simulink model "pneumatiques"  (R2024b)
settings: Solver=VariableStepAuto  StartTime=0.0  StopTime=10.0  RelTol=1e-3
settings Model: Creator=marti  LastModifiedBy=marti

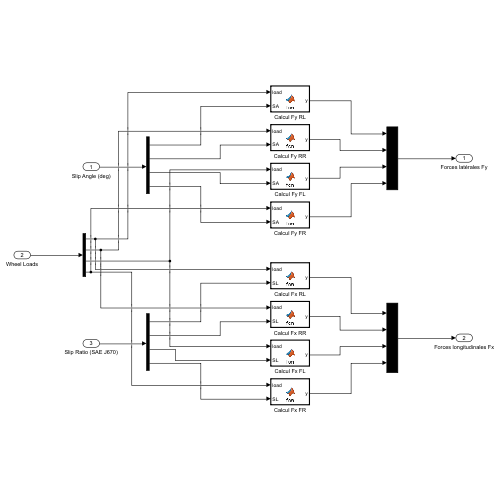
[thumbnail: Simulink's stored preview of the top-level diagram]
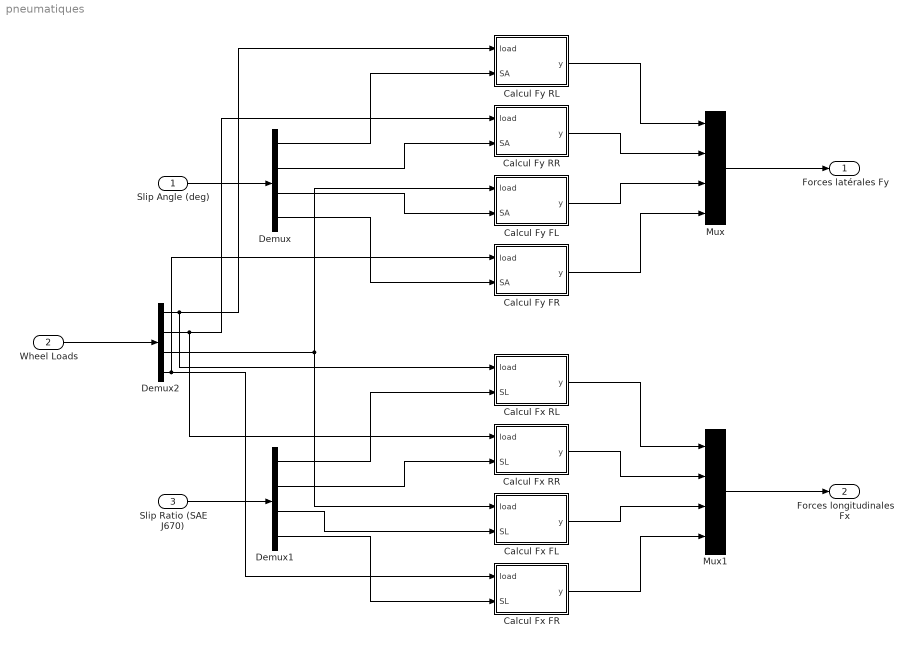
== system pneumatiques ==
  Slip Angle (deg) : Inport
  Wheel Loads : Inport  Port=2
  Slip Ratio (SAE J670) : Inport  Port=3
  Calcul Fx FL : MATLAB Function  TreatAsAtomicUnit=on
  Calcul Fx FR : MATLAB Function  TreatAsAtomicUnit=on
  Calcul Fx RL : MATLAB Function  TreatAsAtomicUnit=on
  Calcul Fx RR : MATLAB Function  TreatAsAtomicUnit=on
  Calcul Fy FL : MATLAB Function  TreatAsAtomicUnit=on
  Calcul Fy FR : MATLAB Function  TreatAsAtomicUnit=on
  Calcul Fy RL : MATLAB Function  TreatAsAtomicUnit=on
  Calcul Fy RR : MATLAB Function  TreatAsAtomicUnit=on
  Demux : Demux
  Demux1 : Demux
  Demux2 : Demux
  Mux : Mux
  Mux1 : Mux
  Forces latérales Fy : Outport
  Forces longitudinales Fx : Outport  Port=2
  wires:
  Slip Angle (deg)/1 -> Demux/1
  Demux/1 -> Calcul Fy RL/2(SA)
  Demux/2 -> Calcul Fy RR/2(SA)
  Demux/3 -> Calcul Fy FL/2(SA)
  Demux/4 -> Calcul Fy FR/2(SA)
  Slip Ratio (SAE J670)/1 -> Demux1/1
  Demux1/2 -> Calcul Fx RR/2(SL)
  Demux1/4 -> Calcul Fx FR/2(SL)
  Demux1/1 -> Calcul Fx RL/2(SL)
  Demux1/3 -> Calcul Fx FL/2(SL)
  Wheel Loads/1 -> Demux2/1
  Demux2/1 -> Calcul Fx RL/1(load), Calcul Fy RL/1(load)
  Demux2/2 -> Calcul Fx RR/1(load), Calcul Fy RR/1(load)
  Demux2/3 -> Calcul Fy FL/1(load), Calcul Fx FL/1(load)
  Demux2/4 -> Calcul Fx FR/1(load), Calcul Fy FR/1(load)
  Calcul Fy RL/1(y) -> Mux/1
  Calcul Fy RR/1(y) -> Mux/2
  Calcul Fy FL/1(y) -> Mux/3
  Calcul Fy FR/1(y) -> Mux/4
  Calcul Fx RL/1(y) -> Mux1/1
  Calcul Fx RR/1(y) -> Mux1/2
  Calcul Fx FL/1(y) -> Mux1/3
  Calcul Fx FR/1(y) -> Mux1/4
  Mux1/1 -> Forces longitudinales Fx/1
  Mux/1 -> Forces latérales Fy/1

== matlab function pneumatiques/Calcul Fy RL ==
  data: load input; y output; SA input
function y = fcn(load,SA)

y = fonction_pacejka_3D_SA(load,SA);
end

== matlab function pneumatiques/Calcul Fy FR ==
  data: load input; y output; SA input
function y = fcn(load,SA)

y = fonction_pacejka_3D_SA(load,SA);
end

== matlab function pneumatiques/Calcul Fy FL ==
  data: load input; y output; SA input
function y = fcn(load,SA)

y = fonction_pacejka_3D_SA(load,SA);
end

== matlab function pneumatiques/Calcul Fx FL ==
  data: load input; y output; SL input
function y = fcn(load,SL)

y = fonction_pacejka_3D_SL(load,SL);
end

== matlab function pneumatiques/Calcul Fx FR ==
  data: load input; y output; SL input
function y = fcn(load,SL)

y = fonction_pacejka_3D_SL(load,SL);
end

== matlab function pneumatiques/Calcul Fx RL ==
  data: load input; y output; SL input
function y = fcn(load,SL)

y = fonction_pacejka_3D_SL(load,SL);
end

== matlab function pneumatiques/Calcul Fx RR ==
  data: load input; y output; SL input
function y = fcn(load,SL)

y = fonction_pacejka_3D_SL(load,SL);
end

== matlab function pneumatiques/Calcul Fy RR ==
  data: load input; y output; SA input
function y = fcn(load,SA)

y = fonction_pacejka_3D_SA(load,SA);
end
